simulink library "TunableDelayBtc"  (R2022b)
settings: Solver=VariableStepAuto  StartTime=0.0  StopTime=10.0  RelTol=1e-3
undefined symbols (not defined in the file or in its folder): Row
libraries: TuneVar x9, HandyTextFile x6, AudioStats x2, $bdroot x2, TOP x2, FeaturePath x2
settings Model: Creator=kl13806  LastModifiedBy=st51187
settings SolverCC: AlgebraicLoopSolver=TrustRegion
settings DebuggingCC: UnconnectedInputMsg=warning  UnconnectedOutputMsg=warning  UnconnectedLineMsg=warning  SFMachineParentedDataDiag=warning
settings ModelReferenceCC: EnableRefExpFcnMdlSchedulingChecks=on
settings RTWCC: DLArmComputeVersion=19.05

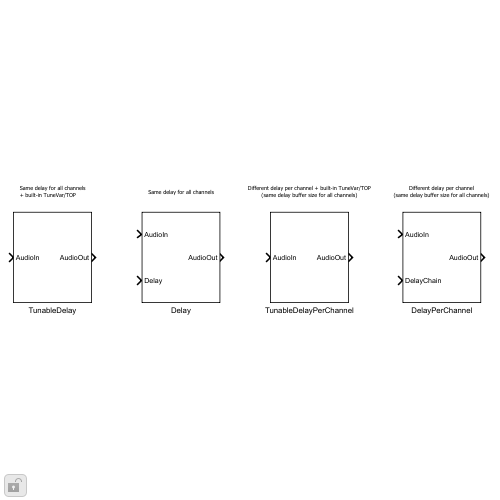
[thumbnail: Simulink's stored preview of the top-level diagram]
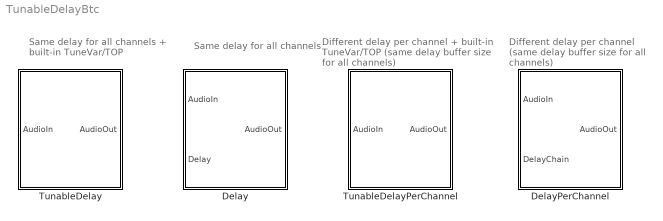
== system TunableDelayBtc ==
  note: Same delay for all channels
      | + built-in TuneVar/TOP
  note: Same delay for all channels
  note: Different delay per channel
      | (same delay buffer size for all channels)
  note: Different delay per channel + built-in TuneVar/TOP
      | (same delay buffer size for all channels)
  Delay : Subsystem  mask(Blocklib Delay){Config=[]}
      mask prompts: Config "DelayConfig"
      mask help:
      | Fixed Alignment Delay
      |
      | This block takes two inputs - delay amount in samples and audio. The same input delay amount is applied to all channels.
      |
      | Note: Please provide a Buffer Alias to the delay in order to access and edit the Header File Name.
      |
      | SHARC+ circular buffer CRL only works for delay amount of type 'int32'.
      mask init:
      | blkh=gcbh;
      | Config=BTConfig.Assert(blkh,Config);
      | TunableDelayMask(gcbh, Config.BufferAlias, Config.HeaderFilename);
      | Config.Validate();
      mask Help:
      | Help on Mask Parameters:
      | 
      | Max Delay (in samples), Frame Size and Number of Channels help determine the circular buffer size. Buffer Alias and Header File Name are useful for memory management in cases where multiple delays are implemented. Both Buffer Alias and Header File Name are reflected in generated code.
      | 
      | Max Delay (in samples): Maximum delay that could be applied to the incoming audio.
      | Frame Size: Frame Size of the incoming audio
      | Number of Channels: Number of channels in incoming audio
      | Buffer Alias: Alias for the circular buffer allocated for this delay instance.
      | Header File Name: Name for header file that specifically manages the delays
  DelayPerChannel : Subsystem  mask(Blocklib DelayPerChannel){Config=[]}
      mask prompts: Config "DelayPerChannelConfig"
      mask help:
      | This block takes two inputs - delay amount in samples and audio. The input delay consists of individual delays for each channel.
      |
      | Note: Please provide a Buffer Alias to the delay in order to access and edit the Header File Name.
      |
      | SHARC+ circular buffer CRL only works for delay amount of type 'int32'.
      mask init:
      | blkh=gcbh;
      | Config=BTConfig.Assert(blkh,Config);
      | TunableDelayMask(gcbh, Config.BufferAlias, Config.HeaderFilename);
      | Config.Validate();
      mask Help:
      | Help on Mask Parameters:
      | 
      | Max Delay (in samples), Frame Size and Number of Channels help determine the circular buffer size. Buffer Alias and Header File Name are useful for memory management in cases where multiple delays are implemented. Both Buffer Alias and Header File Name are reflected in generated code.
      | 
      | Max Delay (in samples): Maximum delay that could be applied to the incoming audio.
      | Frame Size: Frame Size of the incoming audio
      | Number of Channels: Number of channels in incoming audio
      | Buffer Alias: Alias for the circular buffer allocated for this delay instance.
      | Header File Name: Name for header file that specifically manages the delays
      | 
      | For example, if the incoming audio consists of three channels, the incoming delay should be a 1x3 matrix (e.g. [10 20 30]).
      | Each element of delay shall be applied to the corresponding channel fo incoming audio. In the above example, the first input channel would be delayed by 10 samples, the second channel by 20 samples and the third by 30 samples.
  TunableDelay : Subsystem  mask(Blocklib TunableDelay){Config=[], FeatureName=Delay}
      mask prompts: Config "TunableDelayConfig"; FeatureName "Feature path name:"
      mask help:
      | This delay block delays the input by a specified amount in either samples or seconds. The same input delay amount is applied to all channels.
      |
      | Note: Please provide a Buffer Alias to the delay in order to access and edit the Header File Name.
      mask init:
      | blkh=gcbh;
      | Config=BTConfig.Assert(blkh,Config);
      | BTConfig.InitSetFeatureIfPresent(blkh,'FeatureName');
      | Config.Validate();
      mask Help:
      | Help on Mask Parameters:
      | 
      | Max Delay (in samples), Frame Size and Number of Channels help determine the circular buffer size. Buffer Alias and Header File Name are useful for memory management in cases where multiple delays are implemented. Both Buffer Alias and Header File Name are reflected in generated code.
      | 
      | Max Delay (in samples): Maximum delay that could be applied to the incoming audio.
      | Frame Size: Frame Size of the incoming audio
      | Number of Channels: Number of channels in incoming audio
      | Buffer Alias: Alias for the circular buffer allocated for this delay instance.
      | Header File Name: Name for header file that specifically manages the delays
      mask Callback Config: BTConfig.CallbackHideIfPresent(gcbh,{'FeatureName'});
      mask TypeOptions FeatureName: FeaturePath/FeatureName
  TunableDelayPerChannel : Subsystem  mask(Tunable Delay){Config=[], FeatureName=Delay}
      mask prompts: Config "TunableDelayPerChannelConfig"; FeatureName "Feature path name:"
      mask help:
      | This delay block delays the input by a specified amount in either samples or seconds. The same input delay amount is applied to all channels.
      |
      | Note: Please provide a Buffer Alias to the delay in order to access and edit the Header File Name.
      mask init:
      | blkh=gcbh;
      | Config=BTConfig.Assert(blkh,Config);
      | TunableDelayMask(gcbh, Config.BufferAlias, Config.HeaderFilename);
      | BTConfig.InitSetFeatureIfPresent(blkh,'FeatureName');
      | Config.Validate();
      mask Help:
      | Help on Mask Parameters:
      | 
      | Max Delay (in samples), Frame Size and Number of Channels help determine the circular buffer size. Buffer Alias and Header File Name are useful for memory management in cases where multiple delays are implemented. Both Buffer Alias and Header File Name are reflected in generated code.
      | 
      | Max Delay (in samples): Maximum delay that could be applied to the incoming audio.
      | Frame Size: Frame Size of the incoming audio
      | Number of Channels: Number of channels in incoming audio
      | Buffer Alias: Alias for the circular buffer allocated for this delay instance.
      | Header File Name: Name for header file that specifically manages the delays
      mask Callback Config: BTConfig.CallbackHideIfPresent(gcbh,{'FeatureName'});
      mask TypeOptions FeatureName: FeaturePath/FeatureName

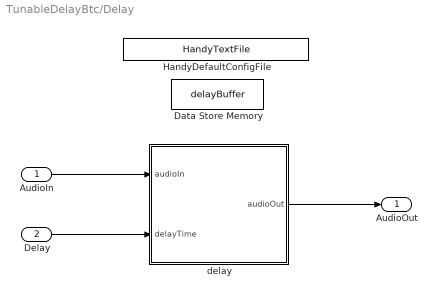
== system TunableDelayBtc/Delay ==
  AudioIn : Inport
  Delay : Inport  Port=2
  Data Store Memory : DataStoreMemory  DataStoreName=delayBuffer  ReadBeforeWriteMsg=warning  WriteAfterWriteMsg=warning  WriteAfterReadMsg=warning  InitialValue=Config.DlgInitialState  ShowAdditionalParam=off  OutDataTypeStr=single
  HandyDefaultConfigFile : HandyTextFile/HandyTextFile  TemplateSource=Config  FileSuffix=Init  OpenDialogOnLoad=off  UseThisBlockName=off  AddGrandParentNamePrefix=off  TheDefaultText=|  ShowInLibBrowser=on
      | % $(FILENAME) Setup model parameters for each "Init" callback (e.g. update diagram)
      | sample_rate_in_hertz = 44100;
      | frame_size = 32;
      | sysin_channel_count = 2;
      settings: SourceProductName=Bose Talaria
  delay : MATLAB Function  TreatAsAtomicUnit=on  mask{maxDelayTime=Config.MaxDelayTime}
  AudioOut : Outport  VectorParamsAs1DForOutWhenUnconnected=off
  wires:
  Delay/1 -> delay/2(delayTime)
  delay/1(audioOut) -> AudioOut/1
  AudioIn/1 -> delay/1(audioIn)

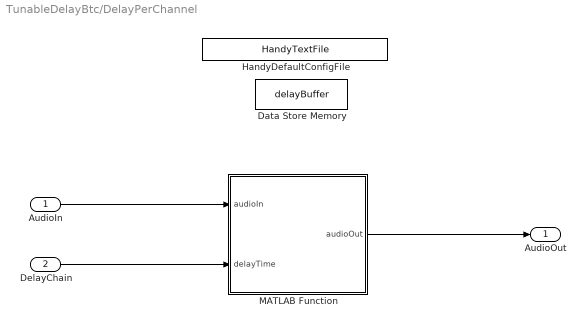
== system TunableDelayBtc/DelayPerChannel ==
  AudioIn : Inport
  DelayChain : Inport  Port=2
  Data Store Memory : DataStoreMemory  DataStoreName=delayBuffer  ReadBeforeWriteMsg=warning  WriteAfterWriteMsg=warning  WriteAfterReadMsg=warning  InitialValue=Config.DlgInitialState  ShowAdditionalParam=off  OutDataTypeStr=single
  HandyDefaultConfigFile : HandyTextFile/HandyTextFile  TemplateSource=Config  FileSuffix=Init  OpenDialogOnLoad=off  UseThisBlockName=off  AddGrandParentNamePrefix=off  TheDefaultText=|  ShowInLibBrowser=on
      | % $(FILENAME) Setup model parameters for each "Init" callback (e.g. update diagram)
      | sample_rate_in_hertz = 44100;
      | frame_size = 32;
      | sysin_channel_count = 2;
      settings: SourceProductName=Bose Talaria
  MATLAB Function : MATLAB Function  TreatAsAtomicUnit=on  mask{maxDelayTime=Config.MaxDelayTime}
  AudioOut : Outport  VectorParamsAs1DForOutWhenUnconnected=off
  wires:
  MATLAB Function/1(audioOut) -> AudioOut/1
  AudioIn/1 -> MATLAB Function/1(audioIn)
  DelayChain/1 -> MATLAB Function/2(delayTime)

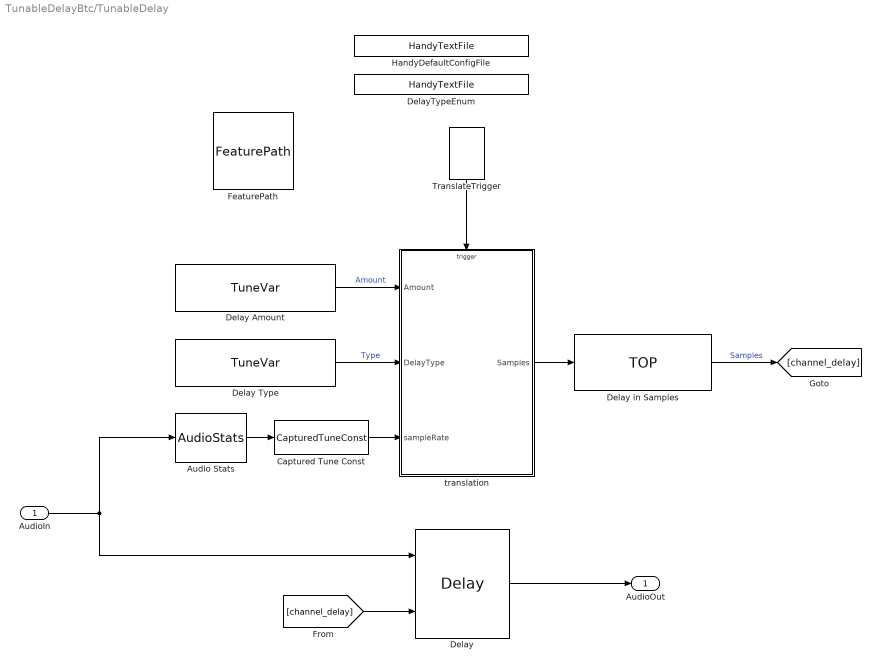
== system TunableDelayBtc/TunableDelay ==
  AudioIn : Inport
  Audio Stats : AudioStats/AudioStats  DoSampleRate=on  TypeSampleRate=Inherit: auto  DoCallRate=off  TypeCallRate=Inherit: auto  DoFrameSize=off  TypeFrameSize=Inherit: auto  DoChannelCount=off  TypeChannelCount=Inherit: auto  DoTaskRateFactor=off  TypeTaskRateFactor=Inherit: auto  MacroNameRoot=AUDIO  MacroNameRootEval='AUDIO'  IsMacroNameEval=off  MacroSampleRate=off  MacroCallRate=off  MacroFrameSize=off  MacroChannelCount=off  MacroTaskRateFactor=off  MacroTaskId=off  ValidateSampleRate=off  ValueSampleRate=[]  ValidateCallRate=off  ValueCallRate=[]  ValidateFrameSize=off  ValueFrameSize=[]  ValidateChannelCount=off  ValueChannelCount=[]  ValidateTaskRateFactor=off  ValueTaskRateFactor=[]
      settings: SourceProductName=Bose Talaria
  Captured Tune Const : TuneVar/CapturedTuneConst  TriggerInit=[610 597 710 633]  Role=Automatic
      settings: SourceProductName=Bose Talaria
  Delay : $bdroot/Delay  Config=Config
      link override Data Store Memory: InitialValue=Config.DlgInitialState
  Delay Amount : TuneVar/TuneVar  TuneName=Amount  SpecifyMaxSize=off  VariableDim=1 (Row)  MaxSize=[1 1]  TunabilityNumber=1  MinValue=[]  MaxValue=[]  TriggerInit=[505 430 675 480]  MaskValue=Config.DefaultDelayAmount
      settings: SourceProductName=Bose Talaria
  Delay Type : TuneVar/TuneVar  Description=|  TuneName=Type  SpecifyMaxSize=off  VariableDim=1 (Row)  MaxSize=[1 1]  TunabilityNumber=1  MinValue=[]  MaxValue=[]  TriggerInit=[505 510 675 560]  MaskValue=int32(Config.DefaultDelayType)
      | Indicates how to interpret the delay amount
      | 1 == InSamples
      | 2 == InMilliseconds
      | (See DelayTypeEnum)
      settings: SourceProductName=Bose Talaria
  Delay in Samples : TOP/TOP  TriggerInit=[930 505 1075 565]  TopName=Samples  DataType=int32  BankNumber=0  PreOverlay=false  PostOverlay=false  Role=Automatic
      settings: SourceProductName=Bose Talaria
  DelayTypeEnum : HandyTextFile/HandyTextFile  TemplateSource=Enum  FileSuffix=Init  OpenDialogOnLoad=off  UseThisBlockName=on  AddGrandParentNamePrefix=off  TheDefaultText=|  ShowInLibBrowser=on
      | % $(FILENAME) Setup model parameters for each "Init" callback (e.g. update diagram)
      | sample_rate_in_hertz = 44100;
      | frame_size = 32;
      | sysin_channel_count = 2;
      settings: SourceProductName=Bose Talaria
  FeaturePath : FeaturePath/FeaturePath  FeatureName=Delay  IsGroup=off  GroupNumber=-1  IsModule=off  TriggerInit=[545 269 630 351]
      settings: SourceProductName=Bose Talaria
  HandyDefaultConfigFile : HandyTextFile/HandyTextFile  TemplateSource=Config  FileSuffix=Init  OpenDialogOnLoad=off  UseThisBlockName=off  AddGrandParentNamePrefix=off  TheDefaultText=|  ShowInLibBrowser=on
      | % $(FILENAME) Setup model parameters for each "Init" callback (e.g. update diagram)
      | sample_rate_in_hertz = 44100;
      | frame_size = 32;
      | sysin_channel_count = 2;
      settings: SourceProductName=Bose Talaria
  TranslateTrigger : TuneVar/TranslateTrigger  TriggerInit=[796 285 834 340]
      settings: SourceProductName=Bose Talaria
  translation : MATLAB Function  TreatAsAtomicUnit=on
  AudioOut : Outport  VectorParamsAs1DForOutWhenUnconnected=off
  wires:
  translation/1(Samples) -> Delay in Samples/1
  [channel_delay] -> Delay/2
  Delay in Samples/1 -> [channel_delay]  "Samples"
  Audio Stats/1 -> Captured Tune Const/1
  Delay/1 -> AudioOut/1
  AudioIn/1 -> Delay/1, Audio Stats/1
  Captured Tune Const/1 -> translation/3(sampleRate)
  Delay Amount/1 -> translation/1(Amount)  "Amount"
  TranslateTrigger/1 -> translation/Trigger
  Delay Type/1 -> translation/2(DelayType)  "Type"

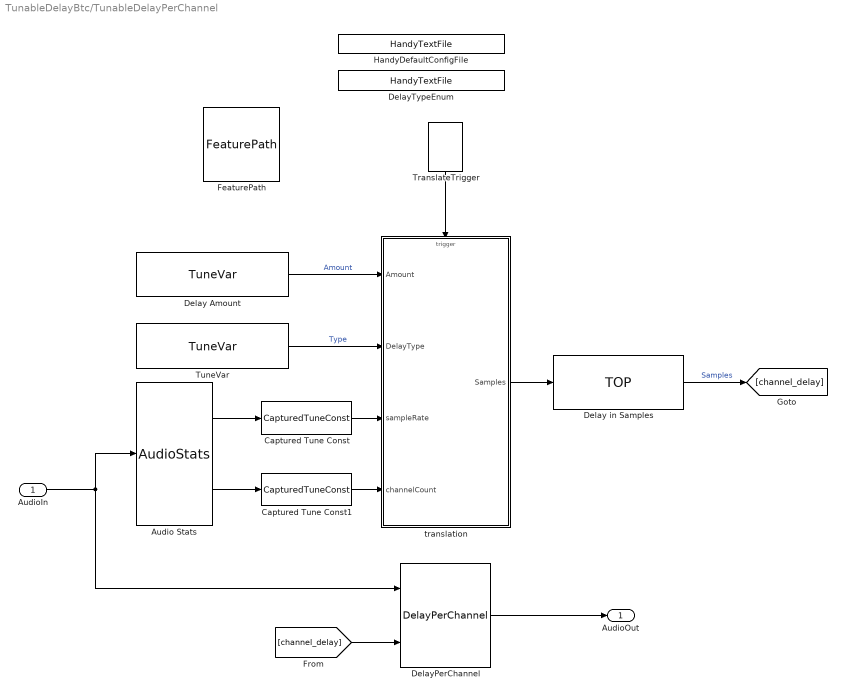
== system TunableDelayBtc/TunableDelayPerChannel ==
  AudioIn : Inport
  Audio Stats : AudioStats/AudioStats  DoSampleRate=on  TypeSampleRate=Inherit: auto  DoCallRate=off  TypeCallRate=Inherit: auto  DoFrameSize=off  TypeFrameSize=Inherit: auto  DoChannelCount=on  TypeChannelCount=Inherit: auto  DoTaskRateFactor=off  TypeTaskRateFactor=Inherit: auto  MacroNameRoot=AUDIO  MacroNameRootEval='AUDIO'  IsMacroNameEval=off  MacroSampleRate=off  MacroCallRate=off  MacroFrameSize=off  MacroChannelCount=off  MacroTaskRateFactor=off  MacroTaskId=off  ValidateSampleRate=off  ValueSampleRate=[]  ValidateCallRate=off  ValueCallRate=[]  ValidateFrameSize=off  ValueFrameSize=[]  ValidateChannelCount=off  ValueChannelCount=[]  ValidateTaskRateFactor=off  ValueTaskRateFactor=[]
      settings: SourceProductName=Bose Talaria
  Captured Tune Const : TuneVar/CapturedTuneConst  TriggerInit=[610 597 710 633]  Role=Automatic
      settings: SourceProductName=Bose Talaria
  Captured Tune Const1 : TuneVar/CapturedTuneConst  TriggerInit=[610 677 710 713]  Role=Automatic
      settings: SourceProductName=Bose Talaria
  Delay Amount : TuneVar/TuneVar  TuneName=Amount  SpecifyMaxSize=off  VariableDim=1 (Row)  MaxSize=[1 1]  TunabilityNumber=1  MinValue=[]  MaxValue=[]  TriggerInit=[470 430 640 480]  MaskValue=Config.DefaultDelayAmount
      settings: SourceProductName=Bose Talaria
  Delay in Samples : TOP/TOP  TriggerInit=[935 545 1080 605]  TopName=Samples  DataType=int32  BankNumber=0  PreOverlay=false  PostOverlay=false  Role=Automatic
      settings: SourceProductName=Bose Talaria
  DelayPerChannel : $bdroot/DelayPerChannel  Config=Config
  DelayTypeEnum : HandyTextFile/HandyTextFile  TemplateSource=Enum  FileSuffix=Init  OpenDialogOnLoad=off  UseThisBlockName=on  AddGrandParentNamePrefix=off  TheDefaultText=|  ShowInLibBrowser=on
      | % $(FILENAME) Setup model parameters for each "Init" callback (e.g. update diagram)
      | sample_rate_in_hertz = 44100;
      | frame_size = 32;
      | sysin_channel_count = 2;
      settings: SourceProductName=Bose Talaria
  FeaturePath : FeaturePath/FeaturePath  FeatureName=Delay  IsGroup=off  GroupNumber=-1  IsModule=off  TriggerInit=[545 269 630 351]
      settings: SourceProductName=Bose Talaria
  HandyDefaultConfigFile : HandyTextFile/HandyTextFile  TemplateSource=Config  FileSuffix=Init  OpenDialogOnLoad=off  UseThisBlockName=off  AddGrandParentNamePrefix=off  TheDefaultText=|  ShowInLibBrowser=on
      | % $(FILENAME) Setup model parameters for each "Init" callback (e.g. update diagram)
      | sample_rate_in_hertz = 44100;
      | frame_size = 32;
      | sysin_channel_count = 2;
      settings: SourceProductName=Bose Talaria
  TranslateTrigger : TuneVar/TranslateTrigger  TriggerInit=[796 285 834 340]
      settings: SourceProductName=Bose Talaria
  TuneVar : TuneVar/TuneVar  TuneName=Type  SpecifyMaxSize=off  VariableDim=1 (Row)  MaxSize=[1 1]  TunabilityNumber=1  MinValue=[]  MaxValue=[]  TriggerInit=[470 510 640 560]  MaskValue=int32(Config.DefaultDelayType)
      settings: SourceProductName=Bose Talaria
  translation : MATLAB Function  TreatAsAtomicUnit=on  mask{maxDelayTime=Config.MaxDelayTime}
  AudioOut : Outport  VectorParamsAs1DForOutWhenUnconnected=off
  wires:
  TranslateTrigger/1 -> translation/Trigger
  Delay Amount/1 -> translation/1(Amount)  "Amount"
  Captured Tune Const/1 -> translation/3(sampleRate)
  AudioIn/1 -> DelayPerChannel/1, Audio Stats/1
  DelayPerChannel/1 -> AudioOut/1
  Audio Stats/1 -> Captured Tune Const/1
  Delay in Samples/1 -> [channel_delay]  "Samples"
  [channel_delay] -> DelayPerChannel/2
  translation/1(Samples) -> Delay in Samples/1
  Captured Tune Const1/1 -> translation/4(channelCount)
  Audio Stats/2 -> Captured Tune Const1/1
  TuneVar/1 -> translation/2(DelayType)  "Type"

== matlab function TunableDelayBtc/TunableDelay/translation ==
  data: Samples output; Amount input; DelayType input; sampleRate input; maxDelayTime parameter
  events: trigger input FUNCTION_CALL_EVENT
function Samples  = fcn(Amount, DelayType, sampleRate, maxDelayTime)

if (DelayType.Value == DelayTypeEnum.InSamples) % delay in samples
    Samples = int32(round(Amount.Value));
else % delay in milliseconds
    Samples = int32(round(Amount.Value * 1e-3 * sampleRate));
end
% Check if the delay is greater than the maximum specified
if Samples > maxDelayTime
    TranslateError('Delay amount cannot be greater than specified max delay');
end

== matlab function TunableDelayBtc/Delay/delay ==
  data: audioIn input; audioOut output; delayTime input size=1; maxDelayTime parameter size=1; delayBuffer data_store_memory
function audioOut = delay(audioIn, delayTime, maxDelayTime)

% Our delayline lives in global variable. We treat as a circular buffer. 
global delayBuffer

% figure out the frame size and channel count
[frameSize, numChannels] = size(audioIn);
frameSize = int32(frameSize);
stateLen = int32(maxDelayTime)+frameSize;
totalLen = int32(stateLen * numChannels);
delayTime = int32(delayTime);
audioOut = coder.nullcopy(audioIn);

% writeIndex points to our current write location in buffer
persistent delayIndex;
if isempty(delayIndex)
    delayIndex = int32(0);
end

% delayBuffer is a circular buffer that holds previous samples

% Write data to delay buffer
bufferIndex = delayIndex;

for channel = 1:numChannels
    
    % Save writeIndex for next channel
    % Instead of writeIndex = bufferIndex, this calls into circindex to set
    % up the registers before any buffer access
    writeIndex = circindex(bufferIndex, int32(0), totalLen);
    
    for sample = 1:frameSize

        % overwrite oldest sample with the current input sample
        delayBuffer(writeIndex + 1) = audioIn(sample, channel);

        % increment write pointer
        writeIndex = circindex(writeIndex, int32(1), totalLen);
    end
    
    % Advance buffer index for next channel
    bufferIndex = circindex(bufferIndex, stateLen, totalLen); 
end

% Reset
bufferIndex = circindex(delayIndex, frameSize, totalLen);
delayIndex = bufferIndex;

% Read samples from delay line
for channel = 1:numChannels
    
    % Setup read pointer
    readIndex = circindex(bufferIndex, -(delayTime+frameSize), totalLen);
    
    for sample = 1:frameSize
       
        % overwrite oldest sample with the current input sample
        audioOut(sample, channel) = delayBuffer(readIndex + 1);
        
        % increment write pointer
        readIndex = circindex(readIndex, int32(1), totalLen);

    end
    
    % Advance buffer index for next channel
    bufferIndex = circindex(bufferIndex, stateLen, totalLen); 
end

end

== matlab function TunableDelayBtc/DelayPerChannel/MATLAB Function ==
  data: audioIn input; audioOut output; delayTime input; maxDelayTime parameter size=1; delayBuffer data_store_memory
function audioOut = delay(audioIn, delayTime, maxDelayTime)

% Our delayline lives in global variable. We treat as a circular buffer. 
global delayBuffer

% figure out the frame size and channel count
[frameSize, numChannels] = size(audioIn);
frameSize = int32(frameSize);
stateLen = int32(maxDelayTime)+frameSize;
totalLen = int32(stateLen * numChannels);
delayTime = int32(delayTime);
audioOut = coder.nullcopy(audioIn);

% writeIndex points to our current write location in buffer
persistent delayIndex;
if isempty(delayIndex)
    delayIndex = int32(0);
end

% delayBuffer is a circular buffer that holds previous samples

% Write data to delay buffer
bufferIndex = delayIndex;

for channel = 1:numChannels
    
    % Save writeIndex for next channel
    % Instead of writeIndex = bufferIndex, this calls into circindex to set
    % up the registers before any buffer access
    writeIndex = circindex(bufferIndex, int32(0), totalLen);
    
    for sample = 1:frameSize

        % overwrite oldest sample with the current input sample
        delayBuffer(writeIndex + 1) = audioIn(sample, channel);

        % increment write pointer
        writeIndex = circindex(writeIndex, int32(1), totalLen);
    end
    
    % Advance buffer index for next channel
    bufferIndex = circindex(bufferIndex, stateLen, totalLen); 
end

% Reset
bufferIndex = circindex(delayIndex, frameSize, totalLen);
delayIndex = bufferIndex;

% Read samples from delay line
for channel = 1:numChannels
    
    % Setup read pointer
    readIndex = circindex(bufferIndex, -(delayTime(channel)+frameSize), totalLen);
    
    for sample = 1:frameSize
       
        % overwrite oldest sample with the current input sample
        audioOut(sample, channel) = delayBuffer(readIndex + 1);
        
        % increment write pointer
        readIndex = circindex(readIndex, int32(1), totalLen);

    end
    
    % Advance buffer index for next channel
    bufferIndex = circindex(bufferIndex, stateLen, totalLen); 
end

end

== matlab function TunableDelayBtc/TunableDelayPerChannel/translation ==
  data: Samples output; Amount input; DelayType input; sampleRate input; channelCount input; maxDelayTime parameter
  events: trigger input FUNCTION_CALL_EVENT
function Samples  = fcn(Amount, DelayType, sampleRate, channelCount, maxDelayTime)

% validate channel count in TuneVar against Delay input
if length(Amount.Value) ~= channelCount
    TranslateError('Mismatch between number of delay tune values and channel count');
end

if (DelayType.Value == DelayTypeEnum.InSamples) % delay in samples
    Samples = int32(round(Amount.Value));
else % delay in milliseconds
    Samples = int32(round(Amount.Value * 1e-3 * sampleRate));
end
% Check if the delay is greater than the maximum specified
if sum(Samples) > maxDelayTime
    TranslateError('Delay amount cannot be greater than specified max delay');
end
